simulink model "sliding_mode_control"  (R2017b)
settings: Solver=FixedStepAuto  StartTime=0.0  StopTime=5.0  RelTol=1e-3
libraries: roblocks x2
settings Model: Creator=root  LastModifiedBy=root

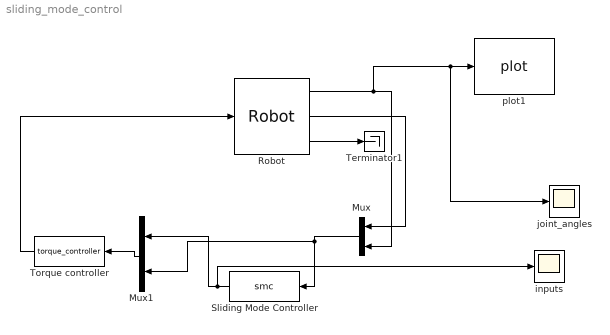
== system sliding_mode_control ==
  Mux : Mux  Inputs=2
  Mux1 : Mux  Inputs=2
  Robot : roblocks/Arm/Robot  robot=twolink  q0=[1 2]
  Sliding Mode Controller : MATLABFcn  MATLABFcn=smc
  Terminator1 : Terminator
  Torque controller : MATLABFcn  MATLABFcn=torque_controller
  inputs : Scope
  joint_angles : Scope
  plot1 : roblocks/Arm/plot  robot=twolink  fps=30  holdplot=on
  wires:
  Robot/3 -> Terminator1/1
  Robot/2 -> Mux/1
  Mux/1 -> Mux1/2, Sliding Mode Controller/1
  Robot/1 -> joint_angles/1, plot1/1, Mux/2
  Torque controller/1 -> Robot/1
  Mux1/1 -> Torque controller/1
  Sliding Mode Controller/1 -> inputs/1, Mux1/1
